simulink model "Exercitiul2"  (R2016a)
settings: Solver=VariableStepDiscrete  StartTime=0.0  StopTime=7200  RelTol=1e-3
undefined symbols (not defined in the file): m, n
settings Model: Creator=Cristina  LastModifiedBy=Cristina

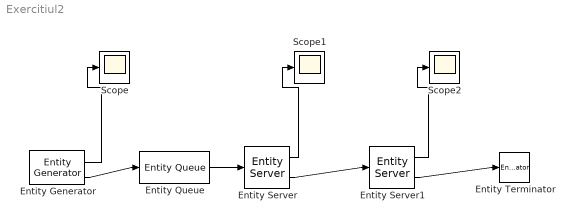
== system Exercitiul2 ==
  Entity Generator : EntityGenerator  OutputPortMessageModes=n,m  TimeSource=MATLAB action  IntergenerationTimeAction=dt = 60 + 120 * rand;  NumberEntitiesDeparted=on  EntityType=Structured  EntityTypeName=Entity
      settings: OutputPortMap=o0,o3
  Entity Queue : EntityQueue  InputPortMessageModes=m  OutputPortMessageModes=m  Capacity=1000
      settings: OutputPortMap=o5
  Entity Server : EntityServer  InputPortMessageModes=m  OutputPortMessageModes=n,m  Capacity=1  ServiceTimeSource=MATLAB action  ServiceTimeAction=dt = 20 + 20 * rand;  AverageWait=on
      settings: OutputPortMap=o4,o9
  Entity Server1 : EntityServer  InputPortMessageModes=m  OutputPortMessageModes=n,m  Capacity=1  ServiceTimeSource=MATLAB action  ServiceTimeAction=dt = 120 + 120 * rand;  AverageWait=on
      settings: OutputPortMap=o4,o9
  Entity Terminator : EntityTerminator  InputPortMessageModes=m
  Scope : Scope
  Scope1 : Scope
  Scope2 : Scope
  wires:
  Entity Server/2 -> Entity Server1/1
  Entity Server1/2 -> Entity Terminator/1
  Entity Queue/1 -> Entity Server/1
  Entity Generator/2 -> Entity Queue/1
  Entity Generator/1 -> Scope/1
  Entity Server/1 -> Scope1/1
  Entity Server1/1 -> Scope2/1
